simulink model "Reglare_cascada_feed_forward"  (R2024b)
settings: Solver=VariableStepAuto  StartTime=0.0  StopTime=1000  RelTol=1e-3  EnableMultiTasking=on
values from neighbouring files (symbols this model uses):
  filtruK = 36.6    [Coeficienti.m]
  h0 = 16.4    [Coeficienti.m]
  hfinal = 19.4    [Coeficienti.m]
  k = 0.046    [Coeficienti.m]
  k1 = 0.624    [Coeficienti.m]
  k2 = -0.015    [Coeficienti.m]
  k3 = -0.0006    [Coeficienti.m]
  keta = 8e-5    (= 8e-05)    [Coeficienti.m]
libraries: slpidlib x2
settings Model: Creator=otudo  LastModifiedBy=receaalex
settings SolverCC: AlgebraicLoopSolver=TrustRegion
settings DataIOCC: ReturnWorkspaceOutputs=off
settings OptimizationCC: LifeSpan=inf
settings DebuggingCC: UnconnectedInputMsg=warning  UnconnectedOutputMsg=warning  UnconnectedLineMsg=warning  SFUnexpectedBacktrackingDiag=warning  SFNoUnconditionalDefaultTransitionDiag=warning  ArithmeticOperatorsInVariantConditions=warning
settings ModelReferenceCC: EnableRefExpFcnMdlSchedulingChecks=on
settings SFSimCC: SimUseLocalCustomCode=off  CustomCodeUndefinedFunction=UseInterfaceOnly
settings RTWCC: RTWUseLocalCustomCode=off  GPUComputeCapability=3.5
settings CodeAppCC: StateflowObjectComments=on
settings GRTTargetCC: TargetLangStandard=C89/C90 (ANSI)
settings ConfigComp: CovMetricSettings=dw  CovSaveCumulativeToWorkspaceVar=on  CovSaveSingleToWorkspaceVar=on  CovExternalEMLEnable=off

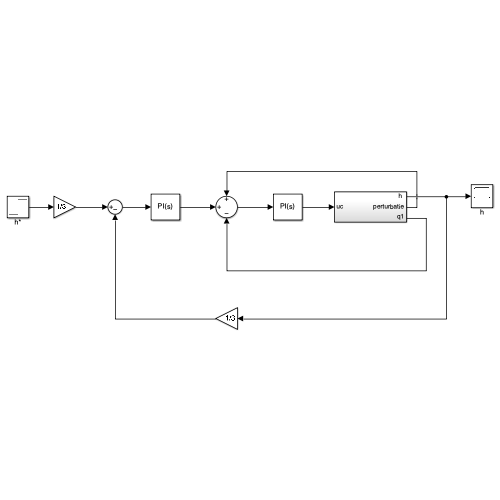
[thumbnail: Simulink's stored preview of the top-level diagram]
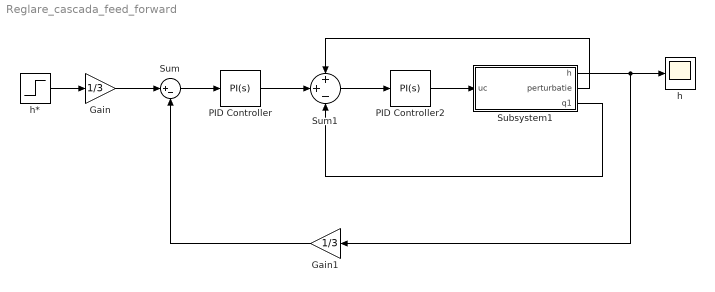
== system Reglare_cascada_feed_forward ==
  Gain : Gain  Gain=1/3
  Gain1 : Gain  Gain=1/3
  PID Controller : slpidlib/PID Controller  Controller=PI  Form=Parallel  TimeDomain=Continuous-time  UseExternalTs=off  SampleTime=-1  IntegratorMethod=Forward Euler  FilterMethod=Forward Euler  ControllerParametersSource=internal  P=19.3424  I=19.3424/300  UseKiTs=off  D=0  UseExternalDerivativeSource=off  N=100  UseFilter=on  TunerSelectOption=Transfer Function Based (PID Tuner App)  InitialConditionSource=internal  InitialConditionForIntegrator=34.4  InitialConditionForFilter=0  DifferentiatorICPrevScaledInput=0  ExternalReset=none  TrackingMode=off  Kt=1  LimitOutput=off  SatLimitsSource=internal  UpperSaturationLimit=inf  LowerSaturationLimit=-inf  LinearizeAsGain=on  AntiWindupMode=none  Kb=1  LimitIntegrator=off  UpperIntegratorSaturationLimit=inf  LowerIntegratorSaturationLimit=-inf  POutMin=[]  POutMax=[]  IOutMin=[]  IOutMax=[]  DOutMin=[]  DOutMax=[]  NOutMin=[]  NOutMax=[]  SumOutMin=[]  SumOutMax=[]  SaturationOutMin=[]  SaturationOutMax=[]  PParamMin=[]  PParamMax=[]  IParamMin=[]  IParamMax=[]  DParamMin=[]  DParamMax=[]  NParamMin=[]  NParamMax=[]  KbParamMin=[]  KbParamMax=[]  KtParamMin=[]  KtParamMax=[]  KbOutMin=[]  KbOutMax=[]  KtOutMin=[]  KtOutMax=[]  IntegratorOutMin=[]  IntegratorOutMax=[]  FilterOutMin=[]  FilterOutMax=[]  SumI1OutMin=[]  SumI1OutMax=[]  SumI2OutMin=[]  SumI2OutMax=[]  SumI3OutMin=[]  SumI3OutMax=[]  SumI4OutMin=[]  SumI4OutMax=[]  SumDOutMin=[]  SumDOutMax=[]  DifferentiatorOutMin=[]  DifferentiatorOutMax=[]  FilterDiffOutCoefMin=[]  FilterDiffOutCoefMax=[]  ReciprocalOutMin=[]  ReciprocalOutMax=[]  SumDenOutMin=[]  SumDenOutMax=[]  SumNumOutMin=[]  SumNumOutMax=[]  DivideOutMin=[]  DivideOutMax=[]  UdiffTsProdOutMin=[]  UdiffTsProdOutMax=[]  NTsProdOutMin=[]  NTsProdOutMax=[]  UintegralTsProdOutMin=[]  UintegralTsProdOutMax=[]  UngainTsProdOutMin=[]  UngainTsProdOutMax=[]  ClampingZeroOutDataTypeStr=Inherit: Inherit via back propagation  ClampingZeroOutMin=[]  ClampingZeroOutMax=[]  FilterDenConstantOutDataTypeStr=Inherit: Inherit via back propagation  FilterDenConstantOutMin=[]  FilterDenConstantOutMax=[]  PCopyOutDataTypeStr=Inherit: Inherit via back propagation  PCopyOutMin=[]  PCopyOutMax=[]  NCopyOutDataTypeStr=Inherit: Inherit via back propagation  NCopyOutMin=[]  NCopyOutMax=[]  IntegratorContinuousStateAttributes=''  IntegratorStateMustResolveToSignalObject=off  IntegratorRTWStateStorageClass=Auto  FilterContinuousStateAttributes=''  FilterStateMustResolveToSignalObject=off  FilterRTWStateStorageClass=Auto  ParallelPVariant=InternalParameters  IdealPVariant=Disabled  IVariant=InternalParameters  DVariant=Disabled  IntegratorVariant=Continuous  SatVariant=Disabled  AWVariant=Passthrough  PCopyVariant=Disabled  TRVariant=Disabled  FdbkBlocksVariant=Forward  IdealPFdbkVariant=Disabled  SatFdbkVariant=Disabled  DerivativeFilterVariant=Disabled  NVariant=Disabled  NCopyVariant=Disabled_SignalSpec  FilterICVariant=Disabled  IntegratorICVariant=InternalICs  ExternalResetVariant=Disabled  TRSumVariant=Passthrough  SumFdbkVariant=Disabled  SumVariant=Sum_PI  TsampFilterVariant=InternalTs  TsampNgainVariant=Passthrough  TsampIntegralVariant=Disabled_SignalSpec  ExternalSaturationOutDataTypeStr=Inherit: Same as second input  DerivativeSourceVariant=Disabled  PreIntVariant=InternalPreInt
  PID Controller2 : slpidlib/PID Controller  Controller=PI  Form=Parallel  TimeDomain=Continuous-time  UseExternalTs=off  SampleTime=-1  IntegratorMethod=Forward Euler  FilterMethod=Forward Euler  ControllerParametersSource=internal  P=0.3  I=0.3/2  UseKiTs=off  D=0  UseExternalDerivativeSource=off  N=100  UseFilter=on  TunerSelectOption=Transfer Function Based (PID Tuner App)  InitialConditionSource=internal  InitialConditionForIntegrator=6  InitialConditionForFilter=0  DifferentiatorICPrevScaledInput=0  ExternalReset=none  TrackingMode=off  Kt=1  LimitOutput=off  SatLimitsSource=internal  UpperSaturationLimit=inf  LowerSaturationLimit=-inf  LinearizeAsGain=on  AntiWindupMode=none  Kb=1  LimitIntegrator=off  UpperIntegratorSaturationLimit=inf  LowerIntegratorSaturationLimit=-inf  POutMin=[]  POutMax=[]  IOutMin=[]  IOutMax=[]  DOutMin=[]  DOutMax=[]  NOutMin=[]  NOutMax=[]  SumOutMin=[]  SumOutMax=[]  SaturationOutMin=[]  SaturationOutMax=[]  PParamMin=[]  PParamMax=[]  IParamMin=[]  IParamMax=[]  DParamMin=[]  DParamMax=[]  NParamMin=[]  NParamMax=[]  KbParamMin=[]  KbParamMax=[]  KtParamMin=[]  KtParamMax=[]  KbOutMin=[]  KbOutMax=[]  KtOutMin=[]  KtOutMax=[]  IntegratorOutMin=[]  IntegratorOutMax=[]  FilterOutMin=[]  FilterOutMax=[]  SumI1OutMin=[]  SumI1OutMax=[]  SumI2OutMin=[]  SumI2OutMax=[]  SumI3OutMin=[]  SumI3OutMax=[]  SumI4OutMin=[]  SumI4OutMax=[]  SumDOutMin=[]  SumDOutMax=[]  DifferentiatorOutMin=[]  DifferentiatorOutMax=[]  FilterDiffOutCoefMin=[]  FilterDiffOutCoefMax=[]  ReciprocalOutMin=[]  ReciprocalOutMax=[]  SumDenOutMin=[]  SumDenOutMax=[]  SumNumOutMin=[]  SumNumOutMax=[]  DivideOutMin=[]  DivideOutMax=[]  UdiffTsProdOutMin=[]  UdiffTsProdOutMax=[]  NTsProdOutMin=[]  NTsProdOutMax=[]  UintegralTsProdOutMin=[]  UintegralTsProdOutMax=[]  UngainTsProdOutMin=[]  UngainTsProdOutMax=[]  ClampingZeroOutDataTypeStr=Inherit: Inherit via back propagation  ClampingZeroOutMin=[]  ClampingZeroOutMax=[]  FilterDenConstantOutDataTypeStr=Inherit: Inherit via back propagation  FilterDenConstantOutMin=[]  FilterDenConstantOutMax=[]  PCopyOutDataTypeStr=Inherit: Inherit via back propagation  PCopyOutMin=[]  PCopyOutMax=[]  NCopyOutDataTypeStr=Inherit: Inherit via back propagation  NCopyOutMin=[]  NCopyOutMax=[]  IntegratorContinuousStateAttributes=''  IntegratorStateMustResolveToSignalObject=off  IntegratorRTWStateStorageClass=Auto  FilterContinuousStateAttributes=''  FilterStateMustResolveToSignalObject=off  FilterRTWStateStorageClass=Auto  ParallelPVariant=InternalParameters  IdealPVariant=Disabled  IVariant=InternalParameters  DVariant=Disabled  IntegratorVariant=Continuous  SatVariant=Disabled  AWVariant=Passthrough  PCopyVariant=Disabled  TRVariant=Disabled  FdbkBlocksVariant=Forward  IdealPFdbkVariant=Disabled  SatFdbkVariant=Disabled  DerivativeFilterVariant=Disabled  NVariant=Disabled  NCopyVariant=Disabled_SignalSpec  FilterICVariant=Disabled  IntegratorICVariant=InternalICs  ExternalResetVariant=Disabled  TRSumVariant=Passthrough  SumFdbkVariant=Disabled  SumVariant=Sum_PI  TsampFilterVariant=InternalTs  TsampNgainVariant=Passthrough  TsampIntegralVariant=Disabled_SignalSpec  ExternalSaturationOutDataTypeStr=Inherit: Same as second input  DerivativeSourceVariant=Disabled  PreIntVariant=InternalPreInt
  Subsystem1 : Subsystem
  Sum : Sum  Inputs=|+-
  Sum1 : Sum  Inputs=++-
  h : Scope
  h* : Step  Before=h0  After=hfinal  SampleTime=0
  wires:
  Sum/1 -> PID Controller/1
  h*/1 -> Gain/1
  Gain/1 -> Sum/1
  Gain1/1 -> Sum/2
  Subsystem1/1("h ") -> Gain1/1, h/1
  Sum1/1 -> PID Controller2/1
  PID Controller2/1 -> Subsystem1/1(uc)
  Subsystem1/3(q1) -> Sum1/3
  PID Controller/1 -> Sum1/2
  Subsystem1/2(perturbatie) -> Sum1/1

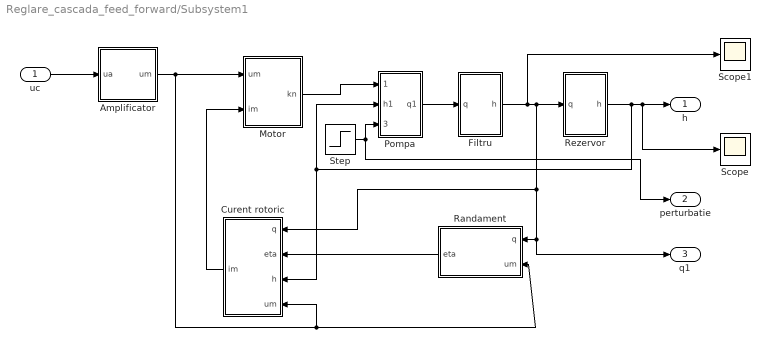
== system Reglare_cascada_feed_forward/Subsystem1 ==
  uc : Inport
  "Amplificator " : Subsystem
  Curent rotoric : Subsystem
  Filtru : Subsystem
  Motor : Subsystem
  Pompa : Subsystem
  Randament : Subsystem
  Rezervor : Subsystem
  Scope : Scope
  Scope1 : Scope
  Step : Step  Time=300  After=k  SampleTime=0
  "h " : Outport
  perturbatie : Outport  Port=2
  q1 : Outport  Port=3
  wires:
  Filtru/1(h) -> Scope1/1, Curent rotoric/1(q), q1/1, Randament/1(q), Rezervor/1(q)
  uc/1 -> "Amplificator "/1(ua)
  Randament/1(eta) -> Curent rotoric/2(eta)
  Rezervor/1(h) -> Curent rotoric/3(h), Pompa/2(h1), Scope/1, "h "/1
  Pompa/1(q1) -> Filtru/1(q)
  Curent rotoric/1(im) -> Motor/2(im)
  "Amplificator "/1(um) -> Curent rotoric/4(um), Randament/2(um), Motor/1(um)
  Motor/1(kn) -> Pompa/1(kn1)
  Step/1 -> perturbatie/1, Pompa/3(perturbatie k)

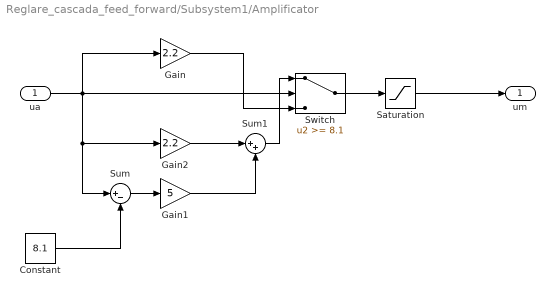
== system Reglare_cascada_feed_forward/Subsystem1/Amplificator  ==
  ua : Inport
  Constant : Constant  Value=8.1
  Gain : Gain  Gain=2.2
  Gain1 : Gain  Gain=5
  Gain2 : Gain  Gain=2.2
  Saturation : Saturate  UpperLimit=22  LowerLimit=0
  Sum : Sum  Inputs=|+-
  Sum1 : Sum  Inputs=|++
  Switch : Switch  Threshold=8.1  SaturateOnIntegerOverflow=off  InputSameDT=off
  um : Outport
  wires:
  Gain/1 -> Switch/3
  Gain1/1 -> Sum1/2
  Switch/1 -> Saturation/1
  Constant/1 -> Sum/2
  Gain2/1 -> Sum1/1
  Sum/1 -> Gain1/1
  Saturation/1 -> um/1
  ua/1 -> Sum/1, Gain2/1, Gain/1, Switch/2
  Sum1/1 -> Switch/1

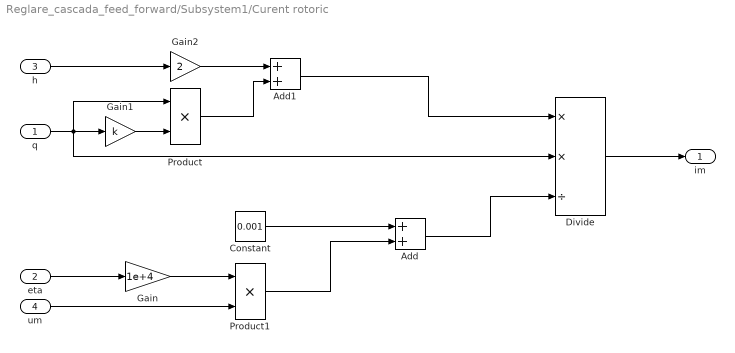
== system Reglare_cascada_feed_forward/Subsystem1/Curent rotoric ==
  q : Inport
  eta : Inport  Port=2
  h : Inport  Port=3
  um : Inport  Port=4
  Add : Sum
  Add1 : Sum
  Constant : Constant  Value=0.001
  Divide : Product  Inputs=**/
  Gain : Gain  Gain=1e+4
  Gain1 : Gain  Gain=k
  Gain2 : Gain  Gain=2
  Product : Product
  Product1 : Product
  im : Outport
  wires:
  Add1/1 -> Divide/1
  Constant/1 -> Add/1
  Add/1 -> Divide/3
  Gain1/1 -> Product/2
  Product/1 -> Add1/2
  um/1 -> Product1/2
  Product1/1 -> Add/2
  Divide/1 -> im/1
  Gain/1 -> Product1/1
  Gain2/1 -> Add1/1
  eta/1 -> Gain/1
  q/1 -> Divide/2, Product/1, Gain1/1
  h/1 -> Gain2/1

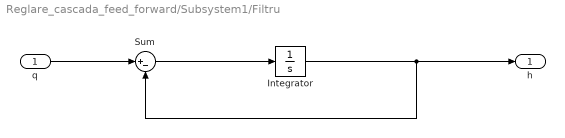
== system Reglare_cascada_feed_forward/Subsystem1/Filtru ==
  q : Inport
  Integrator : Integrator  InitialCondition=filtruK
  Sum : Sum  Inputs=|+-
  h : Outport
  wires:
  Sum/1 -> Integrator/1
  q/1 -> Sum/1
  Integrator/1 -> h/1, Sum/2

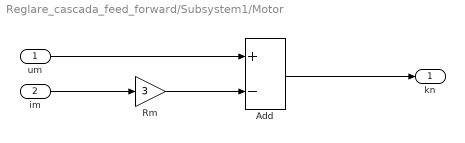
== system Reglare_cascada_feed_forward/Subsystem1/Motor ==
  um : Inport
  im : Inport  Port=2
  Add : Sum  Inputs=+-
  "Rm " : Gain  Gain=3
  kn : Outport
  wires:
  "Rm "/1 -> Add/2
  Add/1 -> kn/1
  um/1 -> Add/1
  im/1 -> "Rm "/1

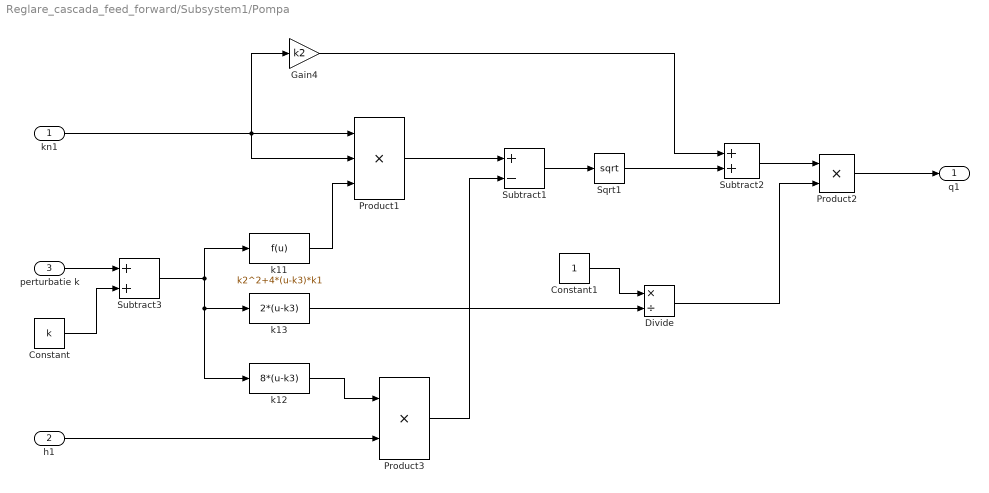
== system Reglare_cascada_feed_forward/Subsystem1/Pompa ==
  kn1 : Inport
  h1 : Inport  Port=2
  perturbatie k : Inport  Port=3
  Constant : Constant  Value=k
  Constant1 : Constant
  Divide : Product  Inputs=*/
  Gain4 : Gain  Gain=k2
  Product1 : Product  Inputs=3
  Product2 : Product
  Product3 : Product
  Sqrt1 : Sqrt
  Subtract1 : Sum  Inputs=+-
  Subtract2 : Sum
  Subtract3 : Sum
  k11 : Fcn  Expr=k2^2+4*(u-k3)*k1
  k12 : Fcn  Expr=8*(u-k3)
  k13 : Fcn  Expr=2*(u-k3)
  q1 : Outport
  wires:
  kn1/1 -> Gain4/1, Product1/1, Product1/2
  Subtract1/1 -> Sqrt1/1
  Gain4/1 -> Subtract2/1
  Sqrt1/1 -> Subtract2/2
  perturbatie k/1 -> Subtract3/1
  Constant/1 -> Subtract3/2
  Product2/1 -> q1/1
  Subtract2/1 -> Product2/1
  Divide/1 -> Product2/2
  Constant1/1 -> Divide/1
  Product1/1 -> Subtract1/1
  h1/1 -> Product3/2
  Product3/1 -> Subtract1/2
  k11/1 -> Product1/3
  Subtract3/1 -> k12/1, k13/1, k11/1
  k12/1 -> Product3/1
  k13/1 -> Divide/2

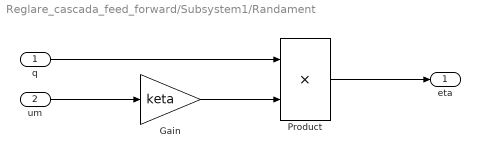
== system Reglare_cascada_feed_forward/Subsystem1/Randament ==
  q : Inport
  um : Inport  Port=2
  Gain : Gain  Gain=keta
  Product : Product
  eta : Outport
  wires:
  Gain/1 -> Product/2
  Product/1 -> eta/1
  q/1 -> Product/1
  um/1 -> Gain/1

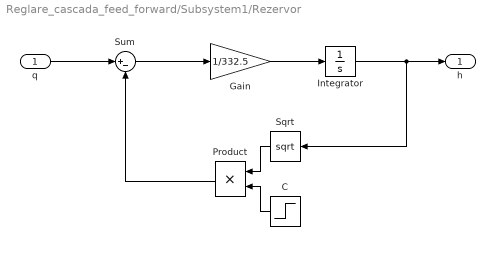
== system Reglare_cascada_feed_forward/Subsystem1/Rezervor ==
  q : Inport
  C : Step  Time=500  Before=9  After=9.2  SampleTime=0
  Gain : Gain  Gain=1/332.5
  Integrator : Integrator  InitialCondition=h0
  Product : Product
  Sqrt : Sqrt
  Sum : Sum  Inputs=|+-
  h : Outport
  wires:
  q/1 -> Sum/1
  Sum/1 -> Gain/1
  Gain/1 -> Integrator/1
  Product/1 -> Sum/2
  C/1 -> Product/2
  Sqrt/1 -> Product/1
  Integrator/1 -> Sqrt/1, h/1
